simulink model "simple_ethercat_master_dc"  (R2018b)
settings: Solver=FixedStepDiscrete  StartTime=0.0  StopTime=100  FixedStep=0.05  RelTol=1e-3  EnableMultiTasking=on
settings Model: FPTRunName=Active  ExtModeTrigDuration=2  Creator=ihout  LastModifiedBy=ihout
settings SolverCC: PositivePriorityOrder=on
settings DataIOCC: LimitDataPoints=on  SaveFormat=Array
settings OptimizationCC: DefaultParameterBehavior=Inlined  ExpressionDepthLimit=2147483647  MaxStackSize=64  SimCompilerOptimization=on
settings DebuggingCC: UnderspecifiedInitializationDetection=Classic  MergeDetectMultiDrivingBlocksExec=none  FcnCallInpInsideContextMsg=warning  AllowSymbolicDim=off  StateNameClashWarn=warning  SFUnexpectedBacktrackingDiag=warning  SFNoUnconditionalDefaultTransitionDiag=warning  SFExecutionAtInitializationDiag=none
settings HardwareCC: UseEmbeddedCoderFeatures=off  UseSimulinkCoderFeatures=off
settings ModelReferenceCC: PropagateSignalLabelsOutOfModel=off
settings SFSimCC: SimUseLocalCustomCode=off
settings RTWCC: SystemTargetFile=sldrt.tlc  MakeCommand="make_rtw OPTS=\" -DWIN32  -D_WINDOWS \""  TemplateMakefile=sldrt.tmf  Description=Simulink Desktop Real-Time  GenerateReport=on  RTWVerbose=off  RTWUseLocalCustomCode=off  Toolchain=GNU GCC Raspberry Pi  BuildConfiguration=Faster Runs  LaunchReport=on  RTWCompilerOptimization=on
settings CodeAppCC: ForceParamTrailComments=on  MaxIdLength=95  OperatorAnnotations=on  StateflowObjectComments=on  MATLABSourceComments=on
settings SimulinkDesktopRealTimeCC: TargetPreCompLibLocation=C:\Program Files\MATLAB\R2018b\toolbox\sldrt\lib\win64  TargetLangStandard=C89/C90 (ANSI)  PreserveStateflowLocalDataDimensions=off
settings ConfigComp: CovMetricSettings=dw  CovHtmlReporting=on  CovSaveCumulativeToWorkspaceVar=on  CovSaveSingleToWorkspaceVar=on  CovExternalEMLEnable=off  CovSFcnEnable=off

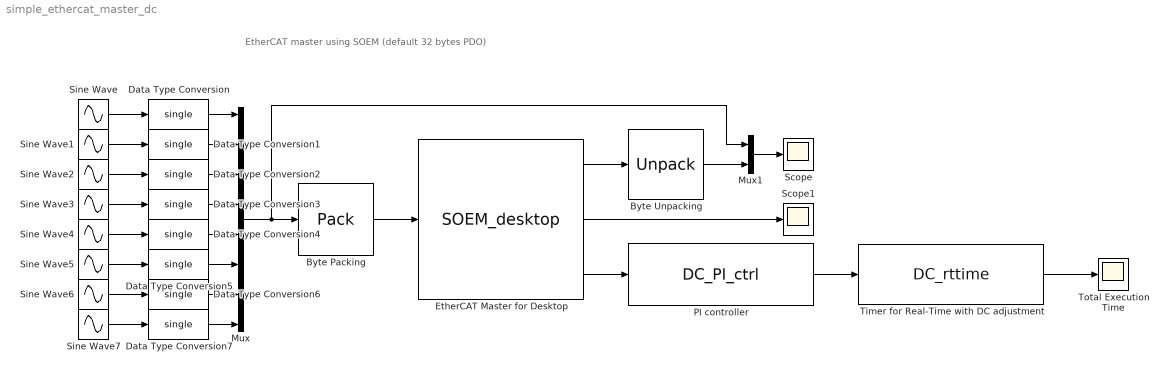
== system simple_ethercat_master_dc ==
  note: EtherCAT master using SOEM (default 32 bytes PDO)
  Byte Packing : S-Function  InitFcn=try, set_param(gcb,'FunctionName','Pack'), end  FunctionName=Pack  SFunctionModules=Pack_wrapper  SFunctionDeploymentMode=off  EnableBusSupport=off  mask(S-Function Builder){}
      mask help: Simulink:masks:SFunctionBuilder_MD
      mask init:
      | val = [[.9  0.75 0.75 1 1 .9 .9 1]',[1 1 0.75 0.75 .9 .9 1 .9]'];try , sys = get_param(gcb,'SfunBuilderFcnName');if isempty(sys), sys = get_param(gcb,'FunctionName'); end,catch, sys = get_param(gcb,'FunctionName'); end
      settings: CopyFcn=set_param(gcbh,'LinkStatus','none')  PreSaveFcn=try, set_param(gcb,'FunctionName','Pack'), end  OpenFcn=sfunctionwizard(gcbh)
      mask Display: plot(val(:,1),val(:,2)),disp(sys), port_label('input',1,'u'), port_label('output',1,'y')
  Byte Unpacking : S-Function  InitFcn=try, set_param(gcb,'FunctionName','Unpack'), end  FunctionName=Unpack  SFunctionModules=Unpack_wrapper  SFunctionDeploymentMode=off  EnableBusSupport=off  mask(S-Function Builder){}
      mask help: Simulink:masks:SFunctionBuilder_MD
      mask init: same as simple_ethercat_master_dc/Byte Packing
      settings: CopyFcn=set_param(gcbh,'LinkStatus','none')  PreSaveFcn=try, set_param(gcb,'FunctionName','Unpack'), end  OpenFcn=sfunctionwizard(gcbh)
      mask Display: plot(val(:,1),val(:,2)),disp(sys), port_label('input',1,'u'), port_label('output',1,'y')
  Data Type Conversion{,1..7} (8 alike) : DataTypeConversion  OutDataTypeStr=single
  EtherCAT Master for Desktop : S-Function  InitFcn=try, set_param(gcb,'FunctionName','SOEM_desktop'), end  FunctionName=SOEM_desktop  Parameters=1,1,0  SFunctionModules=SOEM_desktop_wrapper osal nicdrv oshw ethercatbase ethercatcoe ethercatconfig ethercatdc ethercateoe ethercatfoe ethercatmain ethercatprint ethercatsoe  SFunctionDeploymentMode=off  EnableBusSupport=off  mask(S-Function Builder){}
      mask init: same as simple_ethercat_master_dc/Byte Packing
      settings: CopyFcn=set_param(gcbh,'LinkStatus','none')  PreSaveFcn=try, set_param(gcb,'FunctionName','SOEM_desktop'), end  OpenFcn=sfunctionwizard(gcbh)
      mask Display: plot(val(:,1),val(:,2)),disp(sys), port_label('input',1,'TxPdo'), port_label('output',1,'RxPdo'), port_label('output',2,'State'), port_label('output',3,'DCsyncError')
  Mux : Mux  Inputs=8
  Mux1 : Mux  Inputs=2
  PI controller : S-Function  InitFcn=try, set_param(gcb,'FunctionName','DC_PI_ctrl'), end  FunctionName=DC_PI_ctrl  Parameters=0.2,0.0005  SFunctionModules=DC_PI_ctrl_wrapper  SFunctionDeploymentMode=off  EnableBusSupport=off  mask(S-Function Builder){}
      mask help: Simulink:masks:SFunctionBuilder_MD
      mask init: same as simple_ethercat_master_dc/Byte Packing
      settings: CopyFcn=set_param(gcbh,'LinkStatus','none')  PreSaveFcn=try, set_param(gcb,'FunctionName','DC_PI_ctrl'), end  OpenFcn=sfunctionwizard(gcbh)
      mask Display: plot(val(:,1),val(:,2)),disp(sys), port_label('input',1,'DCsyncError'), port_label('output',1,'DCadjTime')
  Scope : Scope
  Scope1 : Scope
  Sine Wave : Sin  SineType=Sample based  Samples=20  SampleTime=0.05
  Sine Wave1 : Sin  SineType=Sample based  Bias=1  Samples=20  SampleTime=0.05
  Sine Wave2 : Sin  SineType=Sample based  Bias=2  Samples=20  SampleTime=0.05
  Sine Wave3 : Sin  SineType=Sample based  Bias=3  Samples=20  SampleTime=0.05
  Sine Wave4 : Sin  SineType=Sample based  Bias=4  Samples=20  SampleTime=0.05
  Sine Wave5 : Sin  SineType=Sample based  Bias=5  Samples=20  SampleTime=0.05
  Sine Wave6 : Sin  SineType=Sample based  Bias=6  Samples=20  SampleTime=0.05
  Sine Wave7 : Sin  SineType=Sample based  Bias=7  Samples=20  SampleTime=0.05
  Timer for Real-Time with DC adjustment : S-Function  InitFcn=try, set_param(gcb,'FunctionName','DC_rttime'), end  FunctionName=DC_rttime  SFunctionModules=DC_rttime_wrapper  SFunctionDeploymentMode=off  EnableBusSupport=off  mask(S-Function Builder){}
      mask help: Simulink:masks:SFunctionBuilder_MD
      mask init: same as simple_ethercat_master_dc/Byte Packing
      settings: CopyFcn=set_param(gcbh,'LinkStatus','none')  PreSaveFcn=try, set_param(gcb,'FunctionName','DC_rttime'), end  OpenFcn=sfunctionwizard(gcbh)
      mask Display: plot(val(:,1),val(:,2)),disp(sys), port_label('input',1,'DCadjTime'), port_label('output',1,'TET')
  "Total Execution Time " : Scope
  wires:
  Mux/1 -> Mux1/1, Byte Packing/1
  Mux1/1 -> Scope/1
  Data Type Conversion/1 -> Mux/1
  Sine Wave/1 -> Data Type Conversion/1
  EtherCAT Master for Desktop/2 -> Scope1/1
  Byte Packing/1 -> EtherCAT Master for Desktop/1
  EtherCAT Master for Desktop/1 -> Byte Unpacking/1
  Sine Wave7/1 -> Data Type Conversion7/1
  Byte Unpacking/1 -> Mux1/2
  Sine Wave1/1 -> Data Type Conversion1/1
  Data Type Conversion6/1 -> Mux/7
  Data Type Conversion5/1 -> Mux/6
  Sine Wave2/1 -> Data Type Conversion2/1
  Sine Wave4/1 -> Data Type Conversion4/1
  Sine Wave5/1 -> Data Type Conversion5/1
  Sine Wave3/1 -> Data Type Conversion3/1
  Data Type Conversion7/1 -> Mux/8
  Data Type Conversion2/1 -> Mux/3
  EtherCAT Master for Desktop/3 -> PI controller/1
  Data Type Conversion3/1 -> Mux/4
  Sine Wave6/1 -> Data Type Conversion6/1
  Data Type Conversion4/1 -> Mux/5
  Data Type Conversion1/1 -> Mux/2
  Timer for Real-Time with DC adjustment/1 -> "Total Execution Time "/1
  PI controller/1 -> Timer for Real-Time with DC adjustment/1
